simulink model "robustControlNonlinear"  (R2022a)
settings: Solver=VariableStepAuto  StartTime=0.0  StopTime=5  RelTol=1e-3
libraries: simulink x1
settings Model: Creator=Yu  LastModifiedBy=Yu

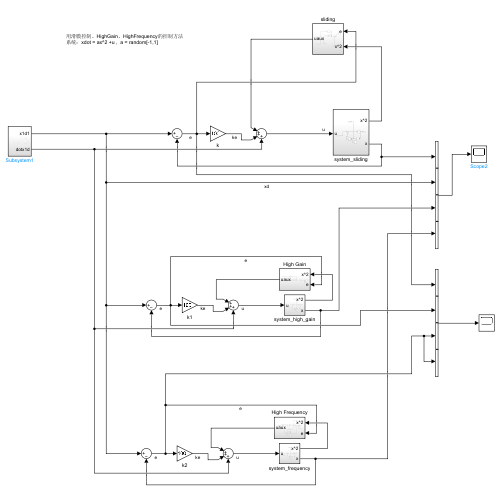
[thumbnail: Simulink's stored preview of the top-level diagram]
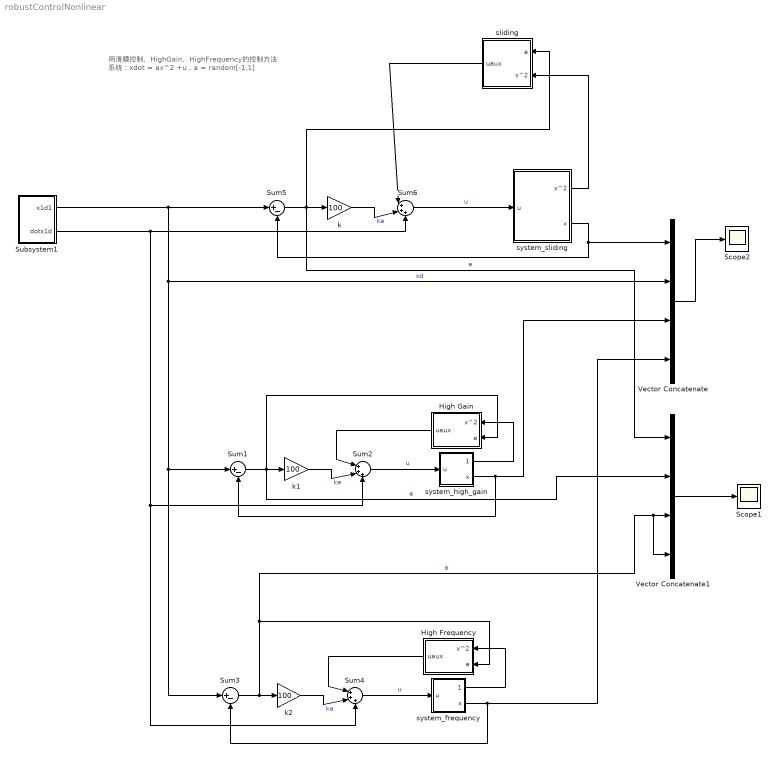
== system robustControlNonlinear ==
  note: 用滑膜控制、HighGain、HighFrequency的控制方法
      | 系统：xdot = ax^2 +u ,  a = random[-1,1]
  High Frequency : Subsystem
  High Gain : Subsystem
  Scope1 : Scope
  Scope2 : Scope
  Subsystem1 : Subsystem
  Sum1 : Sum  Inputs=|+-
  Sum2 : Sum  Inputs=|+++
  Sum3 : Sum  Inputs=|+-
  Sum4 : Sum  Inputs=|+++
  Sum5 : Sum  Inputs=|+-
  Sum6 : Sum  Inputs=|+++
  Vector Concatenate : Concatenate  NumInputs=4
  Vector Concatenate1 : Concatenate  NumInputs=4
  k : Gain  Gain=100
  k1 : Gain  Gain=100
  k2 : Gain  Gain=100
  sliding : Subsystem
  system_frequency : Subsystem
  system_high_gain : Subsystem
  system_sliding : Subsystem
  wires:
  Sum5/1 -> Vector Concatenate1/1, sliding/1(e), k/1  "e"
  k/1 -> Sum6/2  "ke"
  Vector Concatenate/1 -> Scope2/1
  sliding/1(uaux) -> Sum6/1
  system_sliding/2(x) -> Sum5/2, Vector Concatenate/1
  Sum6/1 -> system_sliding/1(u)  "u"
  system_sliding/1(x^2) -> sliding/2(x^2)
  Sum1/1 -> High Gain/2(e), Vector Concatenate1/2, k1/1  "e"
  Sum2/1 -> system_high_gain/1(u)  "u"
  system_high_gain/1(x^2) -> High Gain/1(x^2)
  High Gain/1(uaux) -> Sum2/1
  k1/1 -> Sum2/2  "ke"
  system_high_gain/2(x) -> Vector Concatenate/3, Sum1/2
  system_frequency/1(x^2) -> High Frequency/1(x^2)
  Sum3/1 -> Vector Concatenate1/4, Vector Concatenate1/3, High Frequency/2(e), k2/1  "e"
  Sum4/1 -> system_frequency/1(u)  "u"
  system_frequency/2(x) -> Vector Concatenate/4, Sum3/2
  High Frequency/1(uaux) -> Sum4/1
  Subsystem1/1(x1d1) -> Vector Concatenate/2, Sum1/1, Sum3/1, Sum5/1  "xd"
  k2/1 -> Sum4/2  "ke"
  Subsystem1/2(dotx1d) -> Sum6/3, Sum2/3, Sum4/3
  Vector Concatenate1/1 -> Scope1/1

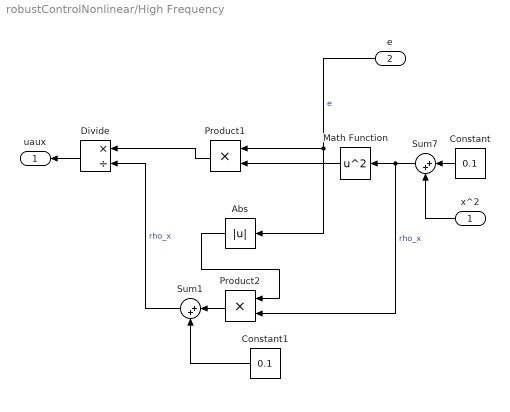
== system robustControlNonlinear/High Frequency ==
  x^2 : Inport
  e : Inport  Port=2
  Abs : Abs  SaturateOnIntegerOverflow=off
  Constant : Constant  Value=0.1
  Constant1 : Constant  Value=0.1
  Divide : Product  Inputs=*/
  Math Function : Math  Operator=square
  Product1 : Product
  Product2 : Product
  Sum1 : Sum  Inputs=|++
  Sum7 : Sum  Inputs=|++
  uaux : Outport
  wires:
  Constant/1 -> Sum7/1
  x^2/1 -> Sum7/2
  Sum7/1 -> Product2/2, Math Function/1  "rho_x"
  Math Function/1 -> Product1/2
  e/1 -> Abs/1, Product1/1  "e"
  Abs/1 -> Product2/1
  Product2/1 -> Sum1/1
  Constant1/1 -> Sum1/2
  Sum1/1 -> Divide/2  "rho_x"
  Product1/1 -> Divide/1
  Divide/1 -> uaux/1

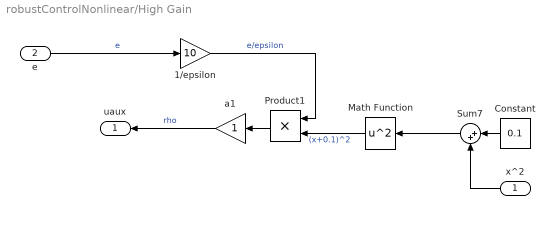
== system robustControlNonlinear/High Gain ==
  x^2 : Inport
  e : Inport  Port=2
  1/epsilon : Gain  Gain=10
  Constant : Constant  Value=0.1
  Math Function : Math  Operator=square
  Product1 : Product
  Sum7 : Sum  Inputs=|++
  a1 : Gain
  uaux : Outport
  wires:
  Constant/1 -> Sum7/1
  a1/1 -> uaux/1  "rho"
  Product1/1 -> a1/1
  x^2/1 -> Sum7/2
  Sum7/1 -> Math Function/1
  Math Function/1 -> Product1/2  "(x+0.1)^2"
  e/1 -> 1/epsilon/1  "e"
  1/epsilon/1 -> Product1/1  "e/epsilon"

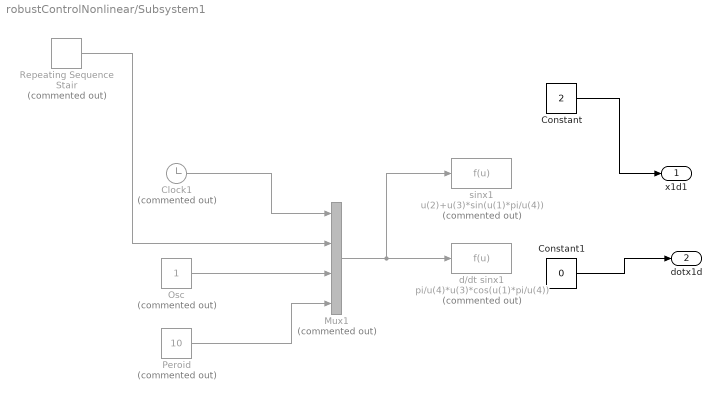
== system robustControlNonlinear/Subsystem1 ==
  Clock1 : Clock  Commented=on
      settings: Decimation=100
  Constant : Constant  Value=2
  Constant1 : Constant  Value=0
  Mux1 : Mux  Commented=on
  Osc : Constant  Commented=on
  Peroid : Constant  Commented=on  Value=10
  Repeating Sequence Stair : simulink/Sources/Repeating Sequence Stair  Commented=on  OutValues=[1 0 1 0 1].'  tsamp=10  OutMin=[]  OutMax=[]  OutDataTypeStr=double  OutputDataTypeScalingMode=double  OutDataType=fixdt(0,8)  ConRadixGroup=Best Precision: Vector-wise  OutScaling=2^-12
  d/dt sinx1 : Fcn  Commented=on  Expr=pi/u(4)*u(3)*cos(u(1)*pi/u(4))
  sinx1 : Fcn  Commented=on  Expr=u(2)+u(3)*sin(u(1)*pi/u(4))
  x1d1 : Outport
  dotx1d : Outport  Port=2
  wires:
  Mux1/1 -> sinx1/1, d/dt sinx1/1
  Repeating Sequence Stair/1 -> Mux1/2
  Clock1/1 -> Mux1/1
  Peroid/1 -> Mux1/4
  Osc/1 -> Mux1/3
  Constant/1 -> x1d1/1
  Constant1/1 -> dotx1d/1

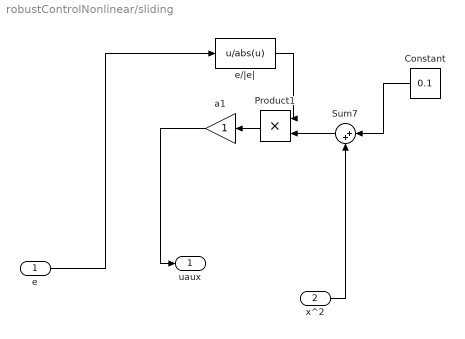
== system robustControlNonlinear/sliding ==
  e : Inport
  x^2 : Inport  Port=2
  Constant : Constant  Value=0.1
  Product1 : Product
  Sum7 : Sum  Inputs=|++
  a1 : Gain
  e/|e| : Fcn  Expr=u/abs(u)
  uaux : Outport
  wires:
  x^2/1 -> Sum7/2
  Constant/1 -> Sum7/1
  Product1/1 -> a1/1
  e/|e|/1 -> Product1/1
  e/1 -> e/|e|/1
  Sum7/1 -> Product1/2
  a1/1 -> uaux/1

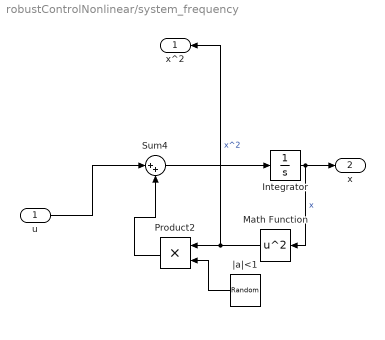
== system robustControlNonlinear/system_frequency ==
  u : Inport
  Integrator : Integrator
  Math Function : Math  Operator=square
  Product2 : Product
  Sum4 : Sum  Inputs=|++
  |a|<1 : UniformRandomNumber  SampleTime=0.1
  x^2 : Outport
  x : Outport  Port=2
  wires:
  u/1 -> Sum4/1
  Product2/1 -> Sum4/2
  Sum4/1 -> Integrator/1
  |a|<1/1 -> Product2/2
  Math Function/1 -> Product2/1, x^2/1  "x^2"
  Integrator/1 -> Math Function/1, x/1  "x"

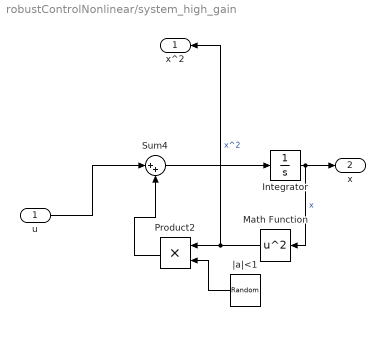
== system robustControlNonlinear/system_high_gain ==
  u : Inport
  Integrator : Integrator
  Math Function : Math  Operator=square
  Product2 : Product
  Sum4 : Sum  Inputs=|++
  |a|<1 : UniformRandomNumber  SampleTime=0.1
  x^2 : Outport
  x : Outport  Port=2
  wires:
  u/1 -> Sum4/1
  Product2/1 -> Sum4/2
  Sum4/1 -> Integrator/1
  |a|<1/1 -> Product2/2
  Math Function/1 -> Product2/1, x^2/1  "x^2"
  Integrator/1 -> Math Function/1, x/1  "x"

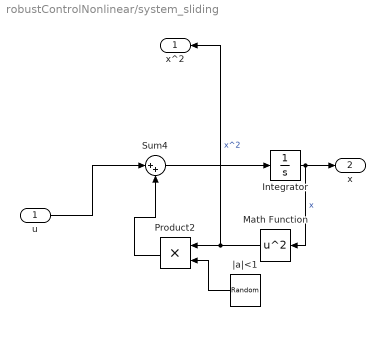
== system robustControlNonlinear/system_sliding ==
  u : Inport
  Integrator : Integrator
  Math Function : Math  Operator=square
  Product2 : Product
  Sum4 : Sum  Inputs=|++
  |a|<1 : UniformRandomNumber  SampleTime=0.1
  x^2 : Outport
  x : Outport  Port=2
  wires:
  Integrator/1 -> x/1, Math Function/1  "x"
  Math Function/1 -> x^2/1, Product2/1  "x^2"
  |a|<1/1 -> Product2/2
  Sum4/1 -> Integrator/1
  Product2/1 -> Sum4/2
  u/1 -> Sum4/1
